simulink model "ms_inter4"  (Simulink 7.3)
settings: Solver=ode45  StartTime=0.0  StopTime=10.0  RelTol=1e-3
settings Model: Creator=sn00632  LastModifiedBy=sn00632

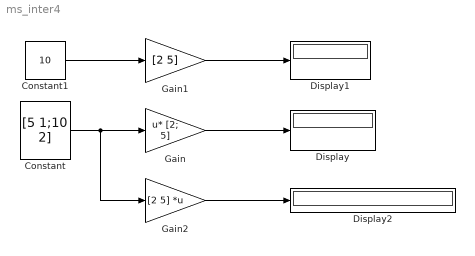
== system ms_inter4 ==
  Constant : Constant  Value=[5 1;10 2]  OutDataType=fixdt(1, 16)  OutScaling=2^0
  Constant1 : Constant  Value=10  OutDataType=fixdt(1, 16)  OutScaling=2^0
  Display : Display
  Display1 : Display
  Display2 : Display
  Gain : Gain  Gain=[2; 5]  Multiplication=Matrix(u*K)  ParameterDataType=fixdt(1, 16)  ParameterScaling=2^0  OutDataType=fixdt(1, 16)  OutScaling=2^0
  Gain1 : Gain  Gain=[2 5]  ParameterDataType=fixdt(1, 16)  ParameterScaling=2^0  OutDataType=fixdt(1, 16)  OutScaling=2^0
  Gain2 : Gain  Gain=[2 5]  Multiplication=Matrix(K*u)  ParameterDataType=fixdt(1, 16)  ParameterScaling=2^0  OutDataType=fixdt(1, 16)  OutScaling=2^0
  wires:
  Gain/1 -> Display/1
  Constant/1 -> Gain/1, Gain2/1
  Gain1/1 -> Display1/1
  Gain2/1 -> Display2/1
  Constant1/1 -> Gain1/1
